simulink model "MPPT_RL"  (R2024b)
settings: Solver=FixedStepAuto  StartTime=0.0  StopTime=9  FixedStep=1e-5  RelTol=1e-3
libraries: spsSeriesRLCBranchLib x24, spsCurrentMeasurementLib x12, spsVoltageMeasurementLib x12, spsMeanLib x8, spsDiodeLib x6, spsMosfetLib x6, spsPVArrayLib x6, spsPWMGeneratorDCDCLib x6, SignalEditorBlockLib x3, spspowerguiLib x3, sps_lib x1
settings Model: Creator=Jatin  LastModifiedBy=Jatin

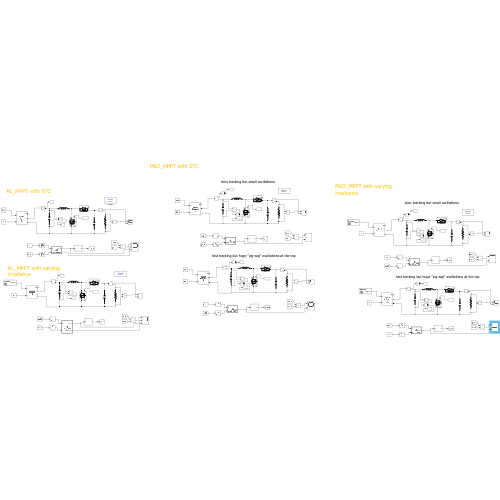
[thumbnail: Simulink's stored preview of the top-level diagram]
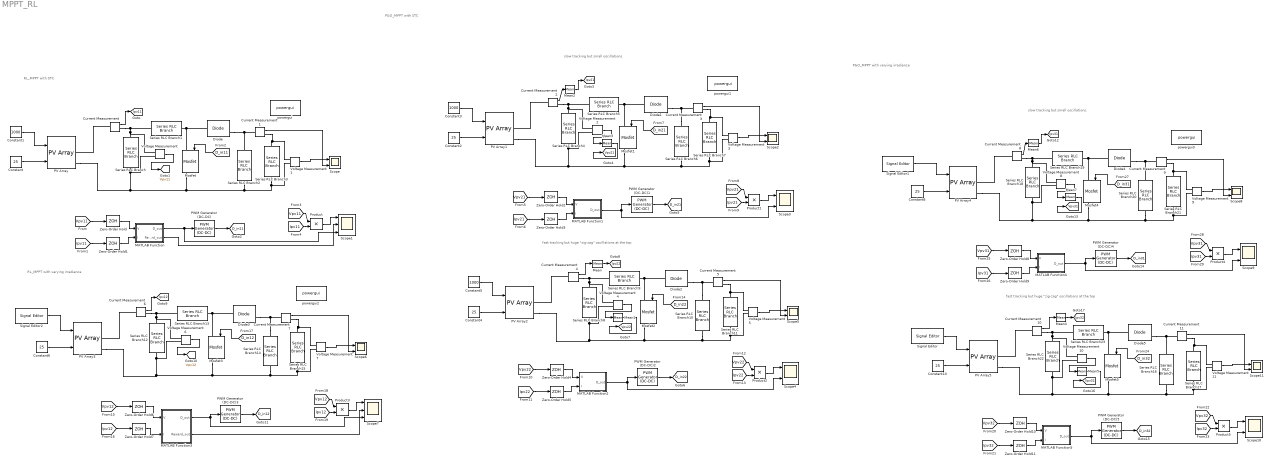
== system MPPT_RL ==
  note: fast tracking but huge "zig-zag" oscillations at the top
  note: slow tracking but small oscillations.
  note: RL_MPPT with STC
  note: P&O_MPPT with STC
  note: RL_MPPT with varying irradiance
  note: P&O_MPPT with varying irradiance
  note: slow tracking but small oscillations.
  note: fast tracking but huge "zig-zag" oscillations at the top
  Constant{,2,4,6,8,10} (6 alike) : Constant  Value=25
  Constant1 : Constant  Value=1000
  Constant3 : Constant  Value=1000
  Constant5 : Constant  Value=1000
  Current Measurement{,1..11} (12 alike) : spsCurrentMeasurementLib/Current Measurement  PhasorSimulation=off  OutputType=Complex  PSBequivalent=0
  Diode{,1..5} (6 alike) : spsDiodeLib/Diode  Ron=0.001  Lon=0  Vf=0  IC=0  UseSnubber=0  Rs=500  Cs=250e-9  Measurements=on
  MATLAB Function : MATLAB Function  TreatAsAtomicUnit=on
  MATLAB Function1 : MATLAB Function  TreatAsAtomicUnit=on
  MATLAB Function2 : MATLAB Function  TreatAsAtomicUnit=on
  MATLAB Function3 : MATLAB Function  TreatAsAtomicUnit=on
  MATLAB Function4 : MATLAB Function  TreatAsAtomicUnit=on
  MATLAB Function5 : MATLAB Function  TreatAsAtomicUnit=on
  Mean{,1..7} (8 alike) : spsMeanLib/Mean  Freq=60  Vinit=0  Ts=0
  Mosfet{,1..5} (6 alike) : spsMosfetLib/Mosfet  Ron=0.1  Lon=0  Rd=0.01  Vfd=0  IC=0  Rs=1e5  Cs=inf  Measurements=on
  PV Array{,1..5} (6 alike) : spsPVArrayLib/PV Array  Npar=1  Nser=1  PlotType=array @ 1000 W/m2 & specified temperatures  S_vec="[ 1000  500  100 ]"  Temp_C_vec="[ 45 25  ]"  ModuleName=User-defined  PlotWhenSelected=off  Pm=59.85  Ncell=60  Voc=21.1  Isc=3.8  Vm=17.1  Im=3.5  beta_Voc_pc=-0.8  alpha_Isc_pc=0.065  beta_Voc=-0.1688  alpha_Isc=0.00247  IL=3.8357  I0=1.4838e-06  nI=0.92819  Rsh=298.3918  Rs=0.10074  RobustModel=off  RobustCellTemperature=313.3991  BAL=on  Tc=1e-6  Tfilter=5e-5
  PWM Generator (DC-DC){,1..5} (6 alike) : spsPWMGeneratorDCDCLib/PWM Generator (DC-DC)  Fsw=5000  Ts=0
  Product{,1..5} (6 alike) : Product
  Scope{,2..6,8..11} (10 alike) : Scope  NumInputPorts=2
  Scope1 : Scope  NumInputPorts=3
  Scope7 : Scope  NumInputPorts=3
  Series RLC Branch{,4,8,12,18,22} (6 alike) : spsSeriesRLCBranchLib/Series RLC Branch  LConnTagsString=__new0  RConnTagsString=__new0  BranchType=C  Resistance=1  Inductance=1e-3  SetiL0=off  InitialCurrent=0  Capacitance=100e-6  Setx0=off  InitialVoltage=0  Measurements=None
  Series RLC Branch{1,5,9,13,19,23} (6 alike) : spsSeriesRLCBranchLib/Series RLC Branch  LConnTagsString=__new0  RConnTagsString=__new0  BranchType=L  Resistance=1  Inductance=3e-3  SetiL0=off  InitialCurrent=0  Capacitance=1e-6  Setx0=off  InitialVoltage=0  Measurements=None
  Series RLC Branch{2,6,10,14,16,20} (6 alike) : spsSeriesRLCBranchLib/Series RLC Branch  LConnTagsString=__new0  RConnTagsString=__new0  BranchType=C  Resistance=1  Inductance=1e-3  SetiL0=off  InitialCurrent=0  Capacitance=470e-6  Setx0=off  InitialVoltage=0  Measurements=None
  Series RLC Branch{3,7,11,15,17,21} (6 alike) : spsSeriesRLCBranchLib/Series RLC Branch  LConnTagsString=__new0  RConnTagsString=__new0  BranchType=R  Resistance=20  Inductance=1e-3  SetiL0=off  InitialCurrent=0  Capacitance=1e-6  Setx0=off  InitialVoltage=0  Measurements=None
  Signal Editor : SignalEditorBlockLib/Signal Editor  FileName=irradiance.mat  ActiveScenario=Scenario  ActiveSignal=Signal 1  IsBus=off  OutputBusObjectStr=Bus: BusObject  SampleTime=0  Interpolate=off  ZeroCross=off  OutputAfterFinalValue=Setting to zero  Unit=inherit  PreserveSignalName=on  ApplySigPropsToAllScenarios=on  ApplySigPropsToAllSignals=off
  Signal Editor1 : SignalEditorBlockLib/Signal Editor  FileName=irradiance.mat  ActiveScenario=Scenario  ActiveSignal=Signal 1  IsBus=off  OutputBusObjectStr=Bus: BusObject  SampleTime=0  Interpolate=off  ZeroCross=off  OutputAfterFinalValue=Setting to zero  Unit=inherit  PreserveSignalName=on  ApplySigPropsToAllScenarios=on  ApplySigPropsToAllSignals=off
  Signal Editor2 : SignalEditorBlockLib/Signal Editor  FileName=irradiance.mat  ActiveScenario=Scenario  ActiveSignal=Signal 1  IsBus=off  OutputBusObjectStr=Bus: BusObject  SampleTime=0  Interpolate=off  ZeroCross=off  OutputAfterFinalValue=Setting to zero  Unit=inherit  PreserveSignalName=on  ApplySigPropsToAllScenarios=on  ApplySigPropsToAllSignals=off
  Voltage Measurement{,1..11} (12 alike) : spsVoltageMeasurementLib/Voltage Measurement  PhasorSimulation=off  OutputType=Complex  PSBequivalent=0
  Zero-Order Hold{,1..11} (12 alike) : ZeroOrderHold  SampleTime=0.01
  powergui : sps_lib/powergui  Priority=1  SimulationMode=Discrete  SampleTime=1e-5  frequency=60  Iterations=50  frequencyindice=0  Pbase=100e6  ErrMax=1e-4  UnitsV=kV  UnitsW=MW  buscounter=0  FunctionMessages=off  echomessages=off  EnableUseOfTLC=off  CurrentSourceSwitches=off  DisableSnubberDevices=off  DisableRonSwitches=off  DisableVfSwitches=off  DisplayEquations=off  AutomaticDiscreteSolvers=off  SolverType=Tustin/Backward Euler (TBE)  Interpol=off  ExternalGateDelay=off  methode=off  Ts=100  x0status=blocks  SPID=on  SwTol=0  HookPort=off  NonlinearTolerance=1e-4  nMaxIteration=100  ContinueOnMaxIteration=off  RestoreLinks=warning  ResistiveCurrentMeasurement=off  Frange=[0:2:500]  Ylog=off  Xlog=on  ShowGrid=off  save=off  variable=ZData  structure=0  ZoomFFT=off  StartTime=0.0  cycles=1  DisplayStyle=1  fundamental=60  FreqAxis=off  MaxFrequency=1000  frequencyindicesteady=1  RmsSteady=1  display=off
  powergui1 : spspowerguiLib/powergui  Priority=1  SimulationMode=Discrete  SampleTime=1e-5  frequency=60  Iterations=50  frequencyindice=0  Pbase=100e6  ErrMax=1e-4  UnitsV=kV  UnitsW=MW  buscounter=0  FunctionMessages=off  echomessages=off  EnableUseOfTLC=off  CurrentSourceSwitches=off  DisableSnubberDevices=off  DisableRonSwitches=off  DisableVfSwitches=off  DisplayEquations=off  AutomaticDiscreteSolvers=off  SolverType=Tustin/Backward Euler (TBE)  Interpol=off  ExternalGateDelay=off  methode=off  Ts=100  x0status=blocks  SPID=on  SwTol=0  HookPort=off  NonlinearTolerance=1e-4  nMaxIteration=100  ContinueOnMaxIteration=off  RestoreLinks=warning  ResistiveCurrentMeasurement=off  Frange=[0:2:500]  Ylog=off  Xlog=on  ShowGrid=off  save=off  variable=ZData  structure=0  ZoomFFT=off  StartTime=0.0  cycles=1  DisplayStyle=1  fundamental=60  FreqAxis=off  MaxFrequency=1000  frequencyindicesteady=1  RmsSteady=1  display=off
  powergui2 : spspowerguiLib/powergui  Priority=1  SimulationMode=Discrete  SampleTime=1e-5  frequency=60  Iterations=50  frequencyindice=0  Pbase=100e6  ErrMax=1e-4  UnitsV=kV  UnitsW=MW  buscounter=0  FunctionMessages=off  echomessages=off  EnableUseOfTLC=off  CurrentSourceSwitches=off  DisableSnubberDevices=off  DisableRonSwitches=off  DisableVfSwitches=off  DisplayEquations=off  AutomaticDiscreteSolvers=off  SolverType=Tustin/Backward Euler (TBE)  Interpol=off  ExternalGateDelay=off  methode=off  Ts=100  x0status=blocks  SPID=on  SwTol=0  HookPort=off  NonlinearTolerance=1e-4  nMaxIteration=100  ContinueOnMaxIteration=off  RestoreLinks=warning  ResistiveCurrentMeasurement=off  Frange=[0:2:500]  Ylog=off  Xlog=on  ShowGrid=off  save=off  variable=ZData  structure=0  ZoomFFT=off  StartTime=0.0  cycles=1  DisplayStyle=1  fundamental=60  FreqAxis=off  MaxFrequency=1000  frequencyindicesteady=1  RmsSteady=1  display=off
  powergui3 : spspowerguiLib/powergui  Priority=1  SimulationMode=Discrete  SampleTime=1e-5  frequency=60  Iterations=50  frequencyindice=0  Pbase=100e6  ErrMax=1e-4  UnitsV=kV  UnitsW=MW  buscounter=0  FunctionMessages=off  echomessages=off  EnableUseOfTLC=off  CurrentSourceSwitches=off  DisableSnubberDevices=off  DisableRonSwitches=off  DisableVfSwitches=off  DisplayEquations=off  AutomaticDiscreteSolvers=off  SolverType=Tustin/Backward Euler (TBE)  Interpol=off  ExternalGateDelay=off  methode=off  Ts=100  x0status=blocks  SPID=on  SwTol=0  HookPort=off  NonlinearTolerance=1e-4  nMaxIteration=100  ContinueOnMaxIteration=off  RestoreLinks=warning  ResistiveCurrentMeasurement=off  Frange=[0:2:500]  Ylog=off  Xlog=on  ShowGrid=off  save=off  variable=ZData  structure=0  ZoomFFT=off  StartTime=0.0  cycles=1  DisplayStyle=1  fundamental=60  FreqAxis=off  MaxFrequency=1000  frequencyindicesteady=1  RmsSteady=1  display=off
  tag scope: D_in11=global, D_in12=global, D_in21=global, D_in22=global, D_in31=global, D_in32=global, Ipv11=global, Ipv12=global, Ipv21=global, Ipv22=global, Ipv31=global, Ipv32=global, Vpv11=global, Vpv12=global, Vpv21=global, Vpv22=global, Vpv31=global, Vpv32=global
  wires:
  Constant/1 -> PV Array/2
  Constant1/1 -> PV Array/1
  Zero-Order Hold/1 -> MATLAB Function/1(V)
  Zero-Order Hold1/1 -> MATLAB Function/2(I)
  Current Measurement/1 -> [Ipv11]
  Voltage Measurement/1 -> [Vpv11]
  [Vpv11] -> Zero-Order Hold/1
  [Ipv11] -> Zero-Order Hold1/1
  MATLAB Function/1(D_out) -> Scope1/3, PWM Generator (DC-DC)/1
  PWM Generator (DC-DC)/1 -> [D_in11]
  [D_in11] -> Mosfet/1
  Voltage Measurement1/1 -> Scope/1
  Current Measurement1/1 -> Scope/2
  [Ipv11] -> Product/2
  [Vpv11] -> Product/1
  Product/1 -> Scope1/1
  MATLAB Function/2(Reward_out) -> Scope1/2
  Current Measurement3/1 -> Scope2/2
  MATLAB Function1/1(D_out) -> Scope3/2, PWM Generator (DC-DC)1/1
  PWM Generator (DC-DC)1/1 -> [D_in21]
  Zero-Order Hold3/1 -> MATLAB Function1/2(I)
  [D_in21] -> Mosfet1/1
  Constant3/1 -> PV Array1/1
  Voltage Measurement3/1 -> Scope2/1
  [Ipv21] -> Zero-Order Hold3/1
  Product1/1 -> Scope3/1
  [Vpv21] -> Zero-Order Hold2/1
  [Ipv21] -> Product1/2
  Constant2/1 -> PV Array1/2
  Zero-Order Hold2/1 -> MATLAB Function1/1(V)
  [Vpv21] -> Product1/1
  Zero-Order Hold4/1 -> MATLAB Function2/1(V)
  [Vpv22] -> Product2/1
  Product2/1 -> Scope4/1
  [Ipv22] -> Product2/2
  Zero-Order Hold5/1 -> MATLAB Function2/2(I)
  PWM Generator (DC-DC)2/1 -> [D_in22]
  MATLAB Function2/1(D_out) -> Scope4/2, PWM Generator (DC-DC)2/1
  Constant4/1 -> PV Array2/2
  Constant5/1 -> PV Array2/1
  Voltage Measurement5/1 -> Scope5/1
  [D_in22] -> Mosfet2/1
  Current Measurement5/1 -> Scope5/2
  [Ipv22] -> Zero-Order Hold5/1
  [Vpv22] -> Zero-Order Hold4/1
  Current Measurement4/1 -> Mean/1
  Mean/1 -> [Ipv22]
  Voltage Measurement4/1 -> Mean1/1
  Mean1/1 -> [Vpv22]
  Current Measurement2/1 -> Mean2/1
  Mean2/1 -> [Ipv21]
  Mean3/1 -> [Vpv21]
  Voltage Measurement2/1 -> Mean3/1
  [Ipv12] -> Zero-Order Hold7/1
  MATLAB Function3/1(D_out) -> PWM Generator (DC-DC)3/1, Scope7/3
  Zero-Order Hold7/1 -> MATLAB Function3/2(I)
  [D_in12] -> Mosfet3/1
  Signal Editor2/1 -> PV Array3/1
  PWM Generator (DC-DC)3/1 -> [D_in12]
  Product3/1 -> Scope7/1
  [Vpv12] -> Zero-Order Hold6/1
  [Vpv12] -> Product3/1
  Current Measurement7/1 -> Scope6/2
  Voltage Measurement6/1 -> [Vpv12]
  Constant6/1 -> PV Array3/2
  [Ipv12] -> Product3/2
  Current Measurement6/1 -> [Ipv12]
  Zero-Order Hold6/1 -> MATLAB Function3/1(V)
  MATLAB Function3/2(Reward_out) -> Scope7/2
  Voltage Measurement7/1 -> Scope6/1
  Mean7/1 -> [Vpv31]
  Zero-Order Hold9/1 -> MATLAB Function4/2(I)
  Product4/1 -> Scope9/1
  Current Measurement9/1 -> Scope8/2
  Voltage Measurement11/1 -> Scope11/1
  Signal Editor/1 -> PV Array5/1
  MATLAB Function4/1(D_out) -> Scope9/2, PWM Generator (DC-DC)4/1
  Mean4/1 -> [Ipv32]
  [Ipv32] -> Product5/2
  PWM Generator (DC-DC)4/1 -> [D_in31]
  [Vpv31] -> Zero-Order Hold8/1
  Constant8/1 -> PV Array4/2
  Zero-Order Hold10/1 -> MATLAB Function5/1(V)
  Mean6/1 -> [Ipv31]
  [Ipv31] -> Zero-Order Hold9/1
  PWM Generator (DC-DC)5/1 -> [D_in32]
  Constant10/1 -> PV Array5/2
  [Vpv32] -> Zero-Order Hold10/1
  Voltage Measurement8/1 -> Mean7/1
  Signal Editor1/1 -> PV Array4/1
  MATLAB Function5/1(D_out) -> Scope10/2, PWM Generator (DC-DC)5/1
  Voltage Measurement10/1 -> Mean5/1
  [Vpv31] -> Product4/1
  [D_in32] -> Mosfet5/1
  Product5/1 -> Scope10/1
  Zero-Order Hold11/1 -> MATLAB Function5/2(I)
  [Vpv32] -> Product5/1
  Current Measurement10/1 -> Mean4/1
  [Ipv31] -> Product4/2
  Current Measurement11/1 -> Scope11/2
  [Ipv32] -> Zero-Order Hold11/1
  Zero-Order Hold8/1 -> MATLAB Function4/1(V)
  Mean5/1 -> [Vpv32]
  [D_in31] -> Mosfet4/1
  Current Measurement8/1 -> Mean6/1
  Voltage Measurement9/1 -> Scope8/1
  connections:
  Series RLC Branch1/LConn1 -- Current Measurement/RConn1 -- Voltage Measurement/LConn1 -- Series RLC Branch/LConn1
  PV Array/RConn2 -- Voltage Measurement1/LConn2 -- Series RLC Branch3/RConn1 -- Series RLC Branch2/RConn1 -- Mosfet/RConn1 -- Voltage Measurement/LConn2 -- Series RLC Branch/RConn1
  Mosfet/LConn1 -- Diode/LConn1 -- Series RLC Branch1/RConn1
  Series RLC Branch3/LConn1 -- Current Measurement1/RConn1 -- Voltage Measurement1/LConn1
  Current Measurement/LConn1 -- PV Array/RConn1
  Diode/RConn1 -- Current Measurement1/LConn1 -- Series RLC Branch2/LConn1
  Series RLC Branch6/LConn1 -- Diode1/RConn1 -- Current Measurement3/LConn1
  Series RLC Branch4/RConn1 -- Voltage Measurement2/LConn2 -- PV Array1/RConn2 -- Voltage Measurement3/LConn2 -- Series RLC Branch7/RConn1 -- Series RLC Branch6/RConn1 -- Mosfet1/RConn1
  Series RLC Branch5/RConn1 -- Mosfet1/LConn1 -- Diode1/LConn1
  Voltage Measurement3/LConn1 -- Series RLC Branch7/LConn1 -- Current Measurement3/RConn1
  Series RLC Branch4/LConn1 -- Series RLC Branch5/LConn1 -- Current Measurement2/RConn1 -- Voltage Measurement2/LConn1
  Current Measurement2/LConn1 -- PV Array1/RConn1
  Voltage Measurement5/LConn1 -- Series RLC Branch11/LConn1 -- Current Measurement5/RConn1
  Series RLC Branch8/RConn1 -- Voltage Measurement4/LConn2 -- PV Array2/RConn2 -- Mosfet2/RConn1 -- Voltage Measurement5/LConn2 -- Series RLC Branch11/RConn1 -- Series RLC Branch10/RConn1
  Series RLC Branch8/LConn1 -- Voltage Measurement4/LConn1 -- Series RLC Branch9/LConn1 -- Current Measurement4/RConn1
  Series RLC Branch9/RConn1 -- Mosfet2/LConn1 -- Diode2/LConn1
  Series RLC Branch10/LConn1 -- Diode2/RConn1 -- Current Measurement5/LConn1
  Current Measurement4/LConn1 -- PV Array2/RConn1
  Series RLC Branch15/RConn1 -- PV Array3/RConn2 -- Voltage Measurement6/LConn2 -- Series RLC Branch12/RConn1 -- Mosfet3/RConn1 -- Series RLC Branch14/RConn1 -- Voltage Measurement7/LConn2
  Series RLC Branch14/LConn1 -- Diode3/RConn1 -- Current Measurement7/LConn1
  Series RLC Branch13/RConn1 -- Mosfet3/LConn1 -- Diode3/LConn1
  Series RLC Branch12/LConn1 -- Voltage Measurement6/LConn1 -- Series RLC Branch13/LConn1 -- Current Measurement6/RConn1
  Voltage Measurement7/LConn1 -- Series RLC Branch15/LConn1 -- Current Measurement7/RConn1
  Current Measurement6/LConn1 -- PV Array3/RConn1
  Diode5/LConn1 -- Mosfet5/LConn1 -- Series RLC Branch23/RConn1
  Current Measurement10/RConn1 -- Series RLC Branch23/LConn1 -- Voltage Measurement10/LConn1 -- Series RLC Branch22/LConn1
  Current Measurement9/RConn1 -- Series RLC Branch21/LConn1 -- Voltage Measurement9/LConn1
  Current Measurement9/LConn1 -- Diode4/RConn1 -- Series RLC Branch20/LConn1
  Series RLC Branch16/RConn1 -- Voltage Measurement11/LConn2 -- Series RLC Branch17/RConn1 -- Mosfet5/RConn1 -- PV Array5/RConn2 -- Voltage Measurement10/LConn2 -- Series RLC Branch22/RConn1
  Current Measurement11/LConn1 -- Diode5/RConn1 -- Series RLC Branch16/LConn1
  Mosfet4/RConn1 -- Voltage Measurement9/LConn2 -- Series RLC Branch21/RConn1 -- Series RLC Branch20/RConn1 -- PV Array4/RConn2 -- Voltage Measurement8/LConn2 -- Series RLC Branch18/RConn1
  Current Measurement11/RConn1 -- Series RLC Branch17/LConn1 -- Voltage Measurement11/LConn1
  Current Measurement8/RConn1 -- Series RLC Branch19/LConn1 -- Voltage Measurement8/LConn1 -- Series RLC Branch18/LConn1
  Diode4/LConn1 -- Mosfet4/LConn1 -- Series RLC Branch19/RConn1
  Current Measurement10/LConn1 -- PV Array5/RConn1
  Current Measurement8/LConn1 -- PV Array4/RConn1

== matlab function MPPT_RL/MATLAB Function1 ==
  data: V input; D_out output; I input
function D_out = PandO_MPPT(V, I)
    persistent D_prev P_prev V_prev Initialized
    
    if isempty(Initialized)
        D_prev = 0.5;       % Initial Duty Cycle
        P_prev = 0;
        V_prev = 0;
        Initialized = 1;
    end
    
    % --- Parameters ---
    % The paper tests two step sizes: 
    % Small = 0.005 (Accurate but slow)
    % Large = 0.05 (Fast but oscillates)
    delta_D = 0.005; 
    
    % --- Calculate Current Power ---
    P = V * I;
    
    % --- P&O Algorithm ---
    dP = P - P_prev;
    dV = V - V_prev;
    
    if dP == 0
        D_new = D_prev; 
    else
        % Logic: If Power increased, keep moving in same direction.
        % If Power decreased, reverse direction
       
        if dP > 0
            if dV > 0
                D_new = D_prev - delta_D; % Move Left (Increase V)
            else
                D_new = D_prev + delta_D; % Move Right (Decrease V)
            end
        else
            if dV > 0
                D_new = D_prev + delta_D;
            else
                D_new = D_prev - delta_D;
            end
        end
    end
    
    % --- Saturation Limits ---
    if D_new > 0.9, D_new = 0.9; end
    if D_new < 0.1, D_new = 0.1; end
    
    % --- Update Memory ---
    D_prev = D_new;
    P_prev = P;
    V_prev = V;
    
    D_out = D_new;
end

== matlab function MPPT_RL/MATLAB Function ==
  data: V input; D_out output; I input; Reward_out output
function [D_out, Reward_out] = RL_MPPT(V, I)
    % RL-MPPT based on Q-Learning [cite: 42, 121]
    
    % --- Persistent Memory (Maintains values between time steps) ---
    persistent Q E_counter D_prev P_prev S_prev A_prev Initialized
    
    % --- Constants from Paper ---
    if isempty(Initialized)
        % State Space: V (0-25V), I (0-4A) [cite: 66, 67]
        % Actions: 5 distinct actions [cite: 78]
        Q = zeros(26, 41, 5); 
        E_counter = 0; 
        D_prev = 0.5; 
        P_prev = 0; 
        S_prev = [1, 1]; % Initial state indices
        A_prev = 3;      % Initial action (index 3 is "No Change")
        Initialized = 1;
    end
    
    % Parameters [cite: 85, 113]
    alpha = 0.1;    % Learning rate
    gamma = 0.9;    % Discount factor
    E_max = 200;    % Max exploration steps
    w_p = 1.5;      % Positive reward weight
    w_n = 1.0;      % Negative reward weight
    
    % Action Space (Change in Duty Cycle) [cite: 78]
    % Actions: 1:-0.05, 2:-0.005, 3:0, 4:+0.005, 5:+0.05
    Actions = [-0.05, -0.005, 0, 0.005, 0.05];
    
    % --- 1. Identify Current State (S_t) ---
    % Voltage: 0-25V with 1V step [cite: 66]
    v_idx = floor(V) + 1;
    if v_idx > 26, v_idx = 26; end
    if v_idx < 1, v_idx = 1; end
    
    % Current: 0-4A with 0.1A step [cite: 67]
    i_idx = floor(I * 10) + 1;
    if i_idx > 41, i_idx = 41; end
    if i_idx < 1, i_idx = 1; end
    
    S_curr = [v_idx, i_idx];
    
    % --- 2. Calculate Reward (r_t) ---
    P_curr = V * I;
    dP = P_curr - P_prev;
    
    % Reward function [cite: 106]
    if dP >= 0
        r = w_p * dP;
    else
        r = w_n * dP;
    end
    
    % --- 3. Update Q-Table (Learning) ---
    % Using Bellman Equation [cite: 175]
    % Q(S,A) = Q(S,A) + alpha * [r + gamma * max(Q(S', :)) - Q(S,A)]
    
    % Max Q value for the CURRENT state (State S')
    max_Q_next = max(Q(v_idx, i_idx, :));
    
    % Update the PREVIOUS state-action pair
    Q_old = Q(S_prev(1), S_prev(2), A_prev);
    Q(S_prev(1), S_prev(2), A_prev) = Q_old + alpha * (r + gamma * max_Q_next - Q_old);
    
    % --- 4. Select Next Action (Policy) ---
    % Exploration vs Exploitation [cite: 179]
    if E_counter < E_max
        % Exploration: Random choice
        A_curr = randi(5);
        E_counter = E_counter + 1;
    else
        % Exploitation: Choose action with max Q-value
        [~, A_curr] = max(Q(v_idx, i_idx, :));
    end
    
    % --- 5. Execute Action ---
    dD = Actions(A_curr);
    D_new = D_prev + dD;
    
    % Saturation (Keep Duty Cycle between 0 and 1)
    if D_new > 0.95, D_new = 0.95; end
    if D_new < 0.05, D_new = 0.05; end
    
    % --- 6. Update History ---
    P_prev = P_curr;
    D_prev = D_new;
    S_prev = S_curr;
    A_prev = A_curr;
    
    D_out = D_new;
    Reward_out=r;
end

== matlab function MPPT_RL/MATLAB Function2 ==
  data: V input; D_out output; I input
function D_out = PandO_MPPT(V, I)
    persistent D_prev P_prev V_prev Initialized
    
    if isempty(Initialized)
        D_prev = 0.5;       % Initial Duty Cycle
        P_prev = 0;
        V_prev = 0;
        Initialized = 1;
    end
    
    % --- Parameters ---
    % The paper tests two step sizes: 
    % Small = 0.005 (Accurate but slow)
    % Large = 0.05 (Fast but oscillates)
    delta_D = 0.02; 
    
    % --- Calculate Current Power ---
    P = V * I;
    
    % --- P&O Algorithm ---
    dP = P - P_prev;
    dV = V - V_prev;
    
    if dP == 0
        D_new = D_prev; 
    else
        % Logic: If Power increased, keep moving in same direction.
        % If Power decreased, reverse direction
       
        if dP > 0
            if dV > 0
                D_new = D_prev - delta_D; % Move Left (Increase V)
            else
                D_new = D_prev + delta_D; % Move Right (Decrease V)
            end
        else
            if dV > 0
                D_new = D_prev + delta_D;
            else
                D_new = D_prev - delta_D;
            end
        end
    end
    
    % --- Saturation Limits ---
    if D_new > 0.9, D_new = 0.9; end
    if D_new < 0.1, D_new = 0.1; end
    
    % --- Update Memory ---
    D_prev = D_new;
    P_prev = P;
    V_prev = V;
    
    D_out = D_new;
end

== matlab function MPPT_RL/MATLAB Function3 ==
  data: V input; D_out output; I input; Reward_out output
function [D_out, Reward_out] = RL_MPPT(V, I)
    % RL-MPPT based on Q-Learning [cite: 42, 121]
    
    % --- Persistent Memory (Maintains values between time steps) ---
    persistent Q E_counter D_prev P_prev S_prev A_prev Initialized
    
    % --- Constants from Paper ---
    if isempty(Initialized)
        % State Space: V (0-25V), I (0-4A) [cite: 66, 67]
        % Actions: 5 distinct actions [cite: 78]
        Q = zeros(26, 41, 5); 
        E_counter = 0; 
        D_prev = 0.5; 
        P_prev = 0; 
        S_prev = [1, 1]; % Initial state indices
        A_prev = 3;      % Initial action (index 3 is "No Change")
        Initialized = 1;
    end
    
    % Parameters [cite: 85, 113]
    alpha = 0.1;    % Learning rate
    gamma = 0.9;    % Discount factor
    E_max = 200;    % Max exploration steps
    w_p = 1.5;      % Positive reward weight
    w_n = 1.0;      % Negative reward weight
    
    % Action Space (Change in Duty Cycle) [cite: 78]
    % Actions: 1:-0.05, 2:-0.005, 3:0, 4:+0.005, 5:+0.05
    Actions = [-0.05, -0.005, 0, 0.005, 0.05];
    
    % --- 1. Identify Current State (S_t) ---
    % Voltage: 0-25V with 1V step [cite: 66]
    v_idx = floor(V) + 1;
    if v_idx > 26, v_idx = 26; end
    if v_idx < 1, v_idx = 1; end
    
    % Current: 0-4A with 0.1A step [cite: 67]
    i_idx = floor(I * 10) + 1;
    if i_idx > 41, i_idx = 41; end
    if i_idx < 1, i_idx = 1; end
    
    S_curr = [v_idx, i_idx];
    
    % --- 2. Calculate Reward (r_t) ---
    P_curr = V * I;
    dP = P_curr - P_prev;
    
    % Reward function [cite: 106]
    if dP >= 0
        r = w_p * dP;
    else
        r = w_n * dP;
    end
    
    % --- 3. Update Q-Table (Learning) ---
    % Using Bellman Equation [cite: 175]
    % Q(S,A) = Q(S,A) + alpha * [r + gamma * max(Q(S', :)) - Q(S,A)]
    
    % Max Q value for the CURRENT state (State S')
    max_Q_next = max(Q(v_idx, i_idx, :));
    
    % Update the PREVIOUS state-action pair
    Q_old = Q(S_prev(1), S_prev(2), A_prev);
    Q(S_prev(1), S_prev(2), A_prev) = Q_old + alpha * (r + gamma * max_Q_next - Q_old);
    
    % --- 4. Select Next Action (Policy) ---
    % Exploration vs Exploitation [cite: 179]
    if E_counter < E_max
        % Exploration: Random choice
        A_curr = randi(5);
        E_counter = E_counter + 1;
    else
        % Exploitation: Choose action with max Q-value
        [~, A_curr] = max(Q(v_idx, i_idx, :));
    end
    
    % --- 5. Execute Action ---
    dD = Actions(A_curr);
    D_new = D_prev + dD;
    
    % Saturation (Keep Duty Cycle between 0 and 1)
    if D_new > 0.95, D_new = 0.95; end
    if D_new < 0.05, D_new = 0.05; end
    
    % --- 6. Update History ---
    P_prev = P_curr;
    D_prev = D_new;
    S_prev = S_curr;
    A_prev = A_curr;
    
    D_out = D_new;
    Reward_out=r;
end

== matlab function MPPT_RL/MATLAB Function4 ==
  data: V input; D_out output; I input
function D_out = PandO_MPPT(V, I)
    persistent D_prev P_prev V_prev Initialized
    
    if isempty(Initialized)
        D_prev = 0.5;       % Initial Duty Cycle
        P_prev = 0;
        V_prev = 0;
        Initialized = 1;
    end
    
    % --- Parameters ---
    % The paper tests two step sizes: 
    % Small = 0.005 (Accurate but slow)
    % Large = 0.05 (Fast but oscillates)
    delta_D = 0.005; 
    
    % --- Calculate Current Power ---
    P = V * I;
    
    % --- P&O Algorithm ---
    dP = P - P_prev;
    dV = V - V_prev;
    
    if dP == 0
        D_new = D_prev; 
    else
        % Logic: If Power increased, keep moving in same direction.
        % If Power decreased, reverse direction
       
        if dP > 0
            if dV > 0
                D_new = D_prev - delta_D; % Move Left (Increase V)
            else
                D_new = D_prev + delta_D; % Move Right (Decrease V)
            end
        else
            if dV > 0
                D_new = D_prev + delta_D;
            else
                D_new = D_prev - delta_D;
            end
        end
    end
    
    % --- Saturation Limits ---
    if D_new > 0.9, D_new = 0.9; end
    if D_new < 0.1, D_new = 0.1; end
    
    % --- Update Memory ---
    D_prev = D_new;
    P_prev = P;
    V_prev = V;
    
    D_out = D_new;
end

== matlab function MPPT_RL/MATLAB Function5 ==
  data: V input; D_out output; I input
function D_out = PandO_MPPT(V, I)
    persistent D_prev P_prev V_prev Initialized
    
    if isempty(Initialized)
        D_prev = 0.5;       % Initial Duty Cycle
        P_prev = 0;
        V_prev = 0;
        Initialized = 1;
    end
    
    % --- Parameters ---
    % The paper tests two step sizes: 
    % Small = 0.005 (Accurate but slow)
    % Large = 0.05 (Fast but oscillates)
    delta_D = 0.02; 
    
    % --- Calculate Current Power ---
    P = V * I;
    
    % --- P&O Algorithm ---
    dP = P - P_prev;
    dV = V - V_prev;
    
    if dP == 0
        D_new = D_prev; 
    else
        % Logic: If Power increased, keep moving in same direction.
        % If Power decreased, reverse direction
       
        if dP > 0
            if dV > 0
                D_new = D_prev - delta_D; % Move Left (Increase V)
            else
                D_new = D_prev + delta_D; % Move Right (Decrease V)
            end
        else
            if dV > 0
                D_new = D_prev + delta_D;
            else
                D_new = D_prev - delta_D;
            end
        end
    end
    
    % --- Saturation Limits ---
    if D_new > 0.9, D_new = 0.9; end
    if D_new < 0.1, D_new = 0.1; end
    
    % --- Update Memory ---
    D_prev = D_new;
    P_prev = P;
    V_prev = V;
    
    D_out = D_new;
end
